simulink model "Simulation"  (R2014a)
settings: Solver=ode45  StartTime=0.0  StopTime=inf  RelTol=1e-3
libraries: vrlib x4, DirectK_Lib x1, InverseK_Lib x1
settings Model: Creator=Cat  LastModifiedBy=Cat

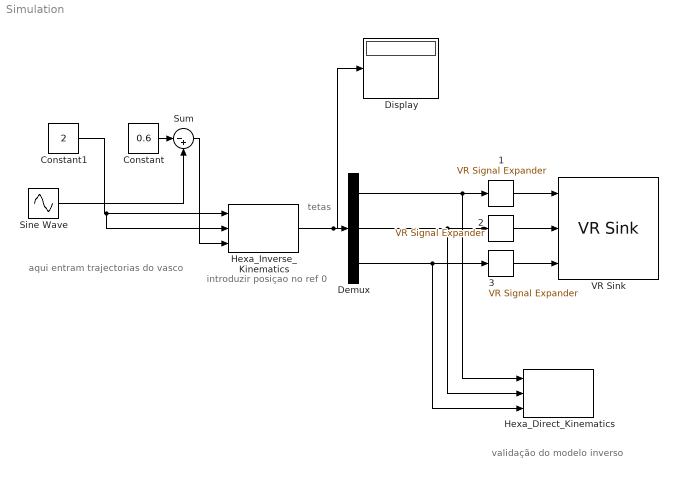
== system Simulation ==
  note: validação do modelo inverso
  note: tetas
  note: introduzir posiçao no ref 0
  note: aqui entram trajectorias do vasco
  1 : vrlib/VR Signal Expander  outwidth=4  outidx=[4]
  2 : vrlib/VR Signal Expander  outwidth=4  outidx=[4]
  3 : vrlib/VR Signal Expander  outwidth=4  outidx=[4]
  Constant : Constant  Value=0.6
  Constant1 : Constant  Value=2
  Demux : Demux  Outputs=3
  Display : Display
  Hexa_Direct_Kinematics : DirectK_Lib/Hexa_Direct_Kinematics
  Hexa_Inverse_Kinematics : InverseK_Lib/Hexa_Inverse_Kinematics
  Sine Wave : Sin  Amplitude=0.3  Frequency=0.7  SampleTime=0
  Sum : Sum  Inputs=|-+
  VR Sink : vrlib/VR Sink  InstantiateOnLoad=on  SampleTime=0.1  ViewEnable=on  RemoteChange=off  RemoteView=off  FieldsWritten=shoulder1transform.rotation.4.1.1.double#Arm1Transform.rotation.4.1.1.double#leg1trasnform.rotation.4.1.1.double  WorldFileName=C:\Users\Cat\Google Drive\Projectos HS\Hexapod\Robotics\VW\vw_old.wrl  AutoView=off  VideoDimensions=[]  AllowVariableSize=off
  wires:
  Hexa_Inverse_Kinematics/1 -> Display/1, Demux/1
  Demux/1 -> 1/1, Hexa_Direct_Kinematics/1
  Demux/2 -> 2/1, Hexa_Direct_Kinematics/2
  Demux/3 -> 3/1, Hexa_Direct_Kinematics/3
  1/1 -> VR Sink/1
  2/1 -> VR Sink/2
  3/1 -> VR Sink/3
  Constant/1 -> Sum/1
  Sum/1 -> Hexa_Inverse_Kinematics/3
  Sine Wave/1 -> Sum/2
  Constant1/1 -> Hexa_Inverse_Kinematics/2, Hexa_Inverse_Kinematics/1
